simulink model "NonLinearModel"  (R2015b)
settings: Solver=VariableStepAuto  StartTime=0.0  StopTime=200  RelTol=1e-3
values from neighbouring files (symbols this model uses):
  Fg = 9.82 * m    (= 4.91)    [Parameters.m]
  Jx = 0.1    [Parameters.m]
  Jy = 0.1    [Parameters.m]
  Jz = 0.2    [Parameters.m]
  kd = 0.0001    [Parameters.m]
  kth = 0.04    [Parameters.m]
  L = 0.16    [Parameters.m]
  m = 0.5    [Parameters.m]
libraries: simulink x4
settings Model: Creator=USUARIO  LastModifiedBy=USUARIO

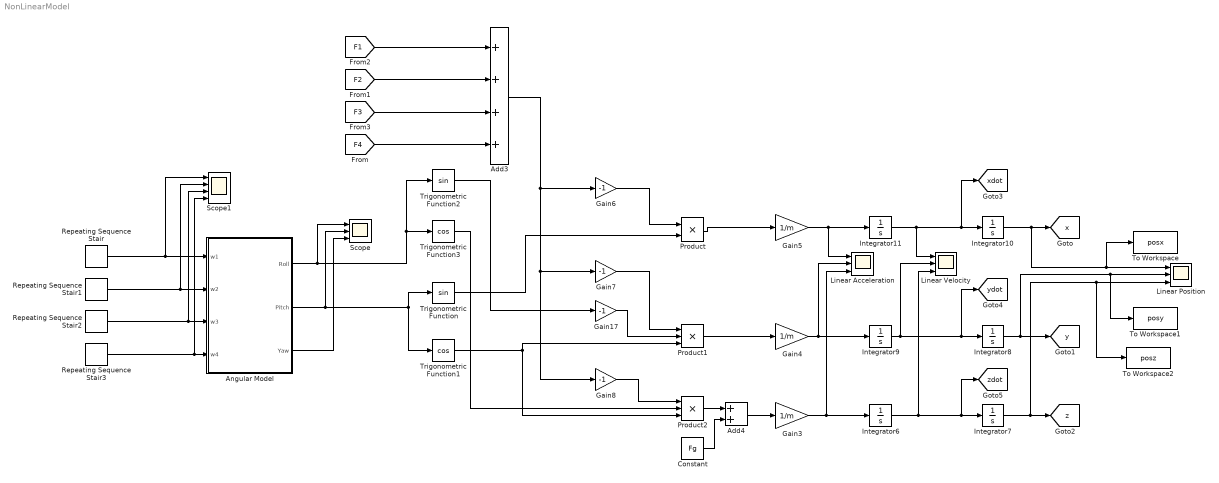
== system NonLinearModel ==
  Add3 : Sum  Inputs=4
  Add4 : Sum  Inputs=2
  Angular Model : Subsystem
  Constant : Constant  Value=Fg
  Gain{6..8,17} (4 alike) : Gain  Gain=-1
  Gain3 : Gain  Gain=1/m
  Gain4 : Gain  Gain=1/m
  Gain5 : Gain  Gain=1/m
  Integrator{6..11} (6 alike) : Integrator
  Linear Acceleration : Scope  NumInputPorts=3
  Linear Position : Scope  NumInputPorts=3
  Linear Velocity : Scope  NumInputPorts=3
  Product : Product
  Product1 : Product  Inputs=3
  Product2 : Product  Inputs=3
  Repeating Sequence Stair{,1..3} (4 alike) : simulink/Sources/Repeating Sequence Stair  OutValues=[3 1 4 2 1].'  tsamp=-1  OutMin=[]  OutMax=[]  OutDataTypeStr=double  OutputDataTypeScalingMode=double  OutDataType=fixdt(0,8)  ConRadixGroup=Best Precision: Vector-wise  OutScaling=2^-12
  Scope : Scope  NumInputPorts=3
  Scope1 : Scope  NumInputPorts=4
  To Workspace : ToWorkspace  VariableName=posx  SampleTime=-1
  To Workspace1 : ToWorkspace  VariableName=posy  SampleTime=-1
  To Workspace2 : ToWorkspace  VariableName=posz  SampleTime=-1
  Trigonometric Function : Trigonometry
  Trigonometric Function1 : Trigonometry  Operator=cos
  Trigonometric Function2 : Trigonometry
  Trigonometric Function3 : Trigonometry  Operator=cos
  tag scope: x=global, xdot=global, y=global, ydot=global, z=global, zdot=global
  wires:
  Product/1 -> Gain5/1
  Product1/1 -> Gain4/1
  Gain5/1 -> Integrator11/1, Linear Acceleration/1
  Gain4/1 -> Integrator9/1, Linear Acceleration/2
  Integrator9/1 -> [ydot], Integrator8/1, Linear Velocity/2
  Integrator11/1 -> [xdot], Integrator10/1, Linear Velocity/1
  Integrator6/1 -> [zdot], Integrator7/1, Linear Velocity/3
  Integrator7/1 -> To Workspace2/1, Linear Position/3, [z]
  Integrator10/1 -> [x], To Workspace/1, Linear Position/1
  Integrator8/1 -> To Workspace1/1, Linear Position/2, [y]
  [F3] -> Add3/3
  [F2] -> Add3/2
  [F1] -> Add3/1
  [F4] -> Add3/4
  Add3/1 -> Gain8/1, Gain7/1, Gain6/1
  Gain6/1 -> Product/1
  Gain7/1 -> Product1/1
  Gain8/1 -> Product2/1
  Product2/1 -> Add4/1
  Add4/1 -> Gain3/1
  Constant/1 -> Add4/2
  Trigonometric Function2/1 -> Gain17/1
  Trigonometric Function/1 -> Product/2
  Gain17/1 -> Product1/2
  Trigonometric Function1/1 -> Product2/3, Product1/3
  Trigonometric Function3/1 -> Product2/2
  Angular Model/1(Roll) -> Scope/1, Trigonometric Function2/1, Trigonometric Function3/1
  Angular Model/2(Pitch) -> Scope/2, Trigonometric Function/1, Trigonometric Function1/1
  Repeating Sequence Stair/1 -> Scope1/1, Angular Model/1(w1)
  Repeating Sequence Stair1/1 -> Scope1/2, Angular Model/2(w2)
  Repeating Sequence Stair2/1 -> Scope1/3, Angular Model/3(w3)
  Repeating Sequence Stair3/1 -> Scope1/4, Angular Model/4(w4)
  Gain3/1 -> Integrator6/1, Linear Acceleration/3
  Angular Model/3(Yaw) -> Scope/3

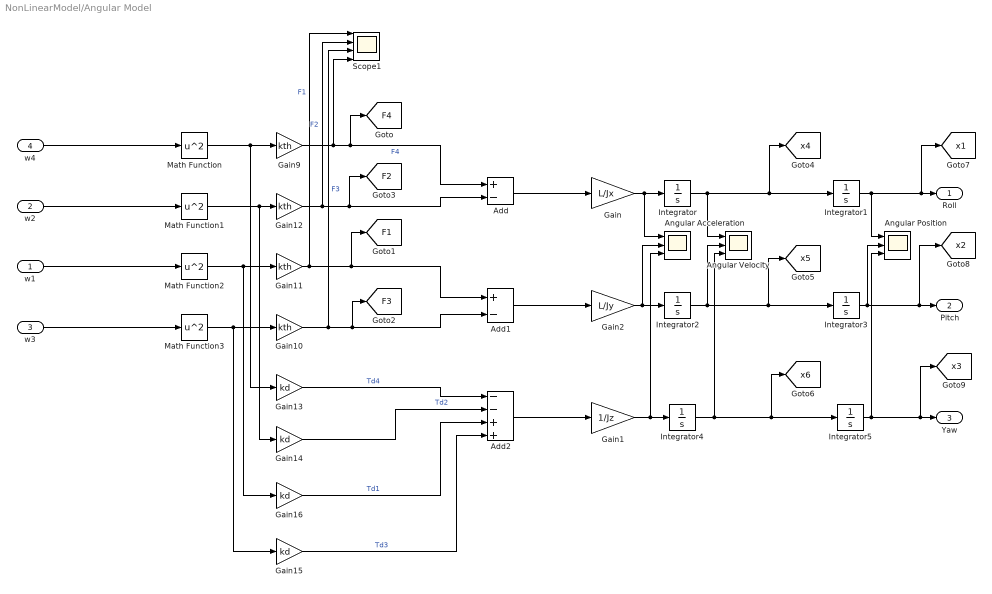
== system NonLinearModel/Angular Model ==
  w1 : Inport
  w2 : Inport  Port=2
  w3 : Inport  Port=3
  w4 : Inport  Port=4
  Add : Sum  Inputs=+-
  Add1 : Sum  Inputs=+-
  Add2 : Sum  Inputs=--++
  Angular Position : Scope  NumInputPorts=3
  Angular Velocity : Scope  NumInputPorts=3
  Angular Acceleration : Scope  NumInputPorts=3
  Gain : Gain  Gain=L/Jx
  Gain1 : Gain  Gain=1/Jz
  Gain{9..12} (4 alike) : Gain  Gain=kth
  Gain{13..16} (4 alike) : Gain  Gain=kd
  Gain2 : Gain  Gain=L/Jy
  Integrator{,1..5} (6 alike) : Integrator
  Math Function{,1..3} (4 alike) : Math  Operator=square  SaturateOnIntegerOverflow=on
  Scope1 : Scope  NumInputPorts=4
  Roll : Outport
  Pitch : Outport  Port=2
  Yaw : Outport  Port=3
  tag scope: F1=global, F2=global, F3=global, F4=global, x1=global, x2=global, x3=global, x4=global, x5=global, x6=global
  wires:
  Gain2/1 -> Angular Acceleration/2, Integrator2/1
  Add2/1 -> Gain1/1
  Gain9/1 -> Scope1/4, [F4], Add/1  "F4"
  Gain14/1 -> Add2/2  "Td2"
  Gain16/1 -> Add2/3  "Td1"
  Gain/1 -> Angular Acceleration/1, Integrator/1
  Integrator/1 -> Angular Velocity/1, Integrator1/1, [x4]
  Integrator1/1 -> [x1], Roll/1, Angular Position/1
  Integrator4/1 -> Angular Velocity/3, [x6], Integrator5/1
  Add/1 -> Gain/1
  Integrator3/1 -> [x2], Pitch/1, Angular Position/2
  Add1/1 -> Gain2/1
  Integrator5/1 -> Angular Position/3, [x3], Yaw/1
  Gain12/1 -> Scope1/2, [F2], Add/2  "F2"
  Gain10/1 -> [F3], Add1/2, Scope1/3  "F3"
  Gain11/1 -> Scope1/1, [F1], Add1/1  "F1"
  Gain13/1 -> Add2/1  "Td4"
  Gain15/1 -> Add2/4  "Td3"
  Integrator2/1 -> Angular Velocity/2, [x5], Integrator3/1
  Gain1/1 -> Angular Acceleration/3, Integrator4/1
  Math Function3/1 -> Gain15/1, Gain10/1
  Math Function2/1 -> Gain16/1, Gain11/1
  Math Function/1 -> Gain13/1, Gain9/1
  Math Function1/1 -> Gain14/1, Gain12/1
  w1/1 -> Math Function2/1
  w2/1 -> Math Function1/1
  w3/1 -> Math Function3/1
  w4/1 -> Math Function/1
